simulink model "ABS_demo"  (R2019a)
settings: Solver=VariableStepAuto  StartTime=0.0  StopTime=15  RelTol=1e-3
undefined symbols (not defined in the file): g, I, m, R, v0
settings Model: Creator=Stephen Kingston  LastModifiedBy=Stephen Kingston

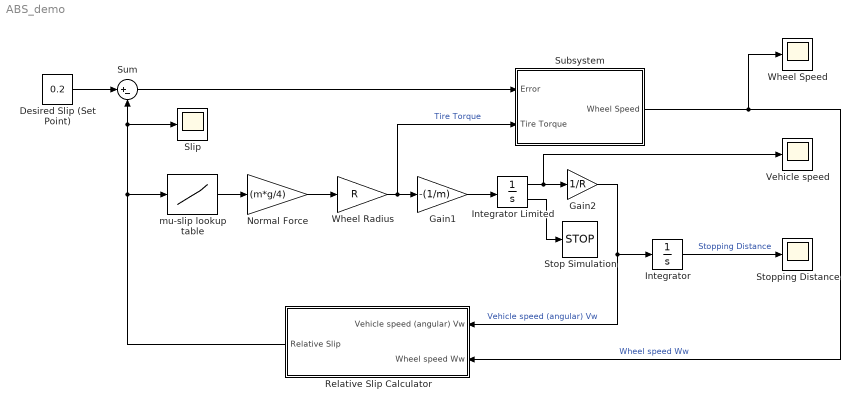
== system ABS_demo ==
  "Desired Slip (Set Point) " : Constant  Value=0.2
  Gain1 : Gain  Gain=-(1/m)
  Gain2 : Gain  Gain=1/R
  Integrator : Integrator
  Integrator Limited : Integrator  InitialCondition=v0  LimitOutput=on  UpperSaturationLimit=1000  LowerSaturationLimit=0  ShowSaturationPort=on
  Normal Force : Gain  Gain=(m*g/4)
  Relative Slip Calculator : Subsystem
  "Slip " : Scope
  Stop Simulation : Stop
  Stopping Distance : Scope
  Subsystem : Subsystem
  Sum : Sum  Inputs=|+-
  Vehicle speed : Scope
  Wheel Radius : Gain  Gain=R
  Wheel Speed : Scope
  mu-slip lookup table : Lookup_n-D  NumberOfTableDimensions=1  BreakpointsForDimension1=[0,0.05,0.1,0.15,0.2,0.25,0.3,0.35,0.4,0.45,0.5,0.55,0.60,0.65,0.70,0.75,0.80,0.85,0.90,0.95,1]  Table=[0,0.4,0.8,0.97,1,0.98,0.96,0.94,0.92,0.9,0.88,0.855,0.83,0.81,0.79,0.77,0.75,0.73,0.72,0.71,0.7]  InternalRulePriority=Speed  RndMeth=Simplest  InputSameDT=on
  wires:
  Sum/1 -> Subsystem/1(Error)
  Wheel Radius/1 -> Gain1/1, Subsystem/2(Tire Torque)  "Tire Torque"
  Gain2/1 -> Relative Slip Calculator/1(Vehicle speed (angular) Vw), Integrator/1  "Vehicle speed (angular) Vw"
  "Desired Slip (Set Point) "/1 -> Sum/1
  mu-slip lookup table/1 -> Normal Force/1
  Normal Force/1 -> Wheel Radius/1
  Gain1/1 -> Integrator Limited/1
  Integrator Limited/1 -> Vehicle speed/1, Gain2/1
  Integrator/1 -> Stopping Distance/1  "Stopping Distance"
  Integrator Limited/2 -> Stop Simulation/1
  Subsystem/1(Wheel Speed) -> Wheel Speed/1, Relative Slip Calculator/2(Wheel speed Ww)  "Wheel speed Ww"
  Relative Slip Calculator/1(Relative Slip) -> "Slip "/1, Sum/2, mu-slip lookup table/1

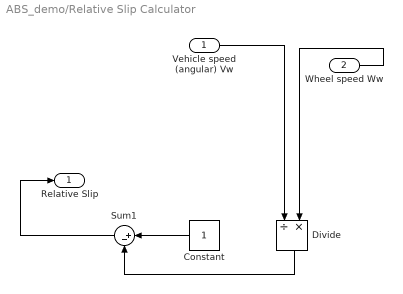
== system ABS_demo/Relative Slip Calculator ==
  Vehicle speed (angular) Vw : Inport
  Wheel speed Ww : Inport  Port=2
  Constant : Constant
  Divide : Product  Inputs=/*
  Sum1 : Sum  Inputs=|+-
  Relative Slip : Outport
  wires:
  Divide/1 -> Sum1/2
  Sum1/1 -> Relative Slip/1
  Constant/1 -> Sum1/1
  Wheel speed Ww/1 -> Divide/2
  Vehicle speed (angular) Vw/1 -> Divide/1

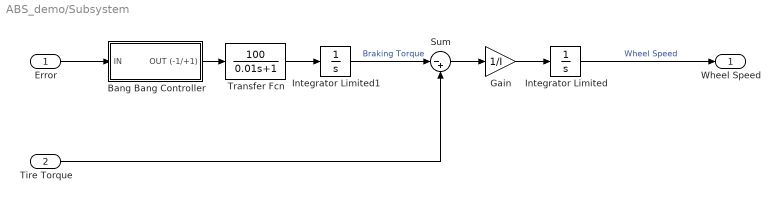
== system ABS_demo/Subsystem ==
  Error : Inport
  Tire Torque : Inport  Port=2
  Bang Bang Controller : Subsystem
  Gain : Gain  Gain=1/I
  Integrator Limited : Integrator  InitialCondition=v0/R  LimitOutput=on  UpperSaturationLimit=1000  LowerSaturationLimit=0
  Integrator Limited1 : Integrator  LimitOutput=on  UpperSaturationLimit=1500  LowerSaturationLimit=0
  Sum : Sum  Inputs=|-+
  Transfer Fcn : TransferFcn  Numerator=[100]  Denominator=[0.01 1]
  Wheel Speed : Outport
  wires:
  Sum/1 -> Gain/1
  Transfer Fcn/1 -> Integrator Limited1/1
  Gain/1 -> Integrator Limited/1
  Integrator Limited/1 -> Wheel Speed/1  "Wheel Speed"
  Integrator Limited1/1 -> Sum/1  "Braking Torque"
  Bang Bang Controller/1(OUT (-1/+1)) -> Transfer Fcn/1
  Tire Torque/1 -> Sum/2
  Error/1 -> Bang Bang Controller/1(IN)

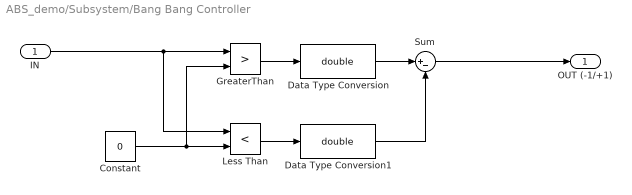
== system ABS_demo/Subsystem/Bang Bang Controller ==
  IN : Inport
  Constant : Constant  Value=0
  Data Type Conversion : DataTypeConversion  OutDataTypeStr=double  RndMeth=Zero
  Data Type Conversion1 : DataTypeConversion  OutDataTypeStr=double  RndMeth=Zero
  GreaterThan : RelationalOperator  Operator=>  OutDataTypeStr=boolean  RndMeth=Simplest
  Less Than : RelationalOperator  Operator=<  OutDataTypeStr=boolean  RndMeth=Simplest
  Sum : Sum  Inputs=|+-
  OUT (-1/+1) : Outport
  wires:
  Sum/1 -> OUT (-1/+1)/1
  Data Type Conversion/1 -> Sum/1
  Constant/1 -> GreaterThan/2, Less Than/2
  IN/1 -> Less Than/1, GreaterThan/1
  Data Type Conversion1/1 -> Sum/2
  GreaterThan/1 -> Data Type Conversion/1
  Less Than/1 -> Data Type Conversion1/1
